simulink model "trojBez"  (Simulink 7.5)
settings: Solver=ode45  StartTime=0.0  StopTime=40.0  RelTol=1e-3
settings Model: Creator=168092  LastModifiedBy=TC

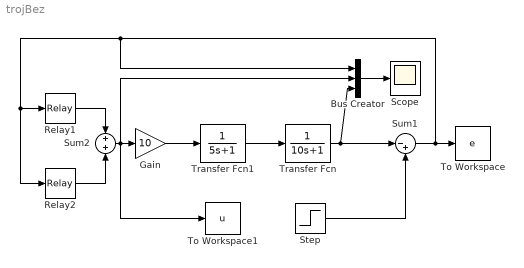
== system trojBez ==
  Bus Creator : BusCreator  Inputs=3
  Gain : Gain  Gain=10  ParameterDataType=fixdt(1, 16)  ParameterScaling=2^0  OutDataType=fixdt(1, 16)  OutScaling=2^0
  Relay1 : Relay  OnSwitchValue=0.1  OffSwitchValue=0.1  OutDataType=fixdt(1, 16)  OutScaling=2^0
  Relay2 : Relay  OnSwitchValue=-0.1  OffSwitchValue=-0.1  OnOutputValue=0  OffOutputValue=-1  OutDataType=fixdt(1, 16)  OutScaling=2^0
  Scope : Scope
      settings: TickLabels=on  TimeRange=30  YMin=0  YMax=1  SampleInput=on
  Step : Step  Time=0  After=2.5  SampleTime=0
  Sum1 : Sum  Inputs=|-+  OutDataType=fixdt(1, 16)  OutScaling=2^0
  Sum2 : Sum  OutDataType=fixdt(1, 16)  OutScaling=2^0
  To Workspace : ToWorkspace  VariableName=e  SampleTime=-1  SaveFormat=Structure
  To Workspace1 : ToWorkspace  VariableName=u  SampleTime=-1  SaveFormat=Structure
  Transfer Fcn : TransferFcn  Denominator=[10 1]
  Transfer Fcn1 : TransferFcn  Denominator=[5 1]
  wires:
  Transfer Fcn/1 -> Sum1/1, Bus Creator/3
  Gain/1 -> Transfer Fcn1/1
  Transfer Fcn1/1 -> Transfer Fcn/1
  Bus Creator/1 -> Scope/1
  Sum1/1 -> To Workspace/1, Bus Creator/1, Relay2/1, Relay1/1
  Step/1 -> Sum1/2
  Sum2/1 -> Bus Creator/2, Gain/1, To Workspace1/1
  Relay1/1 -> Sum2/1
  Relay2/1 -> Sum2/2
